simulink model "CLSfixed"  (R2024b)
settings: Solver=FixedStepAuto  StartTime=0.0  StopTime=3000  FixedStep=stepsize  RelTol=1e-3
undefined symbols (not defined in the file or in its folder): AVI, cfg_length, LRI, pNode_length, pPath_length, PVARP, stepsize, URI, VRP
libraries: Libs_unified x311
(part 4 of 4)

== matlab function CLSfixed/Plotting ==
  data: t input; u input
function fcn(t,u)
%coder.extrinsic('evalin')
coder.extrinsic('updateGUIplots')
fun = 'updateGUIplots';
updateGUIplots(t,u)
%feval(fun,t,u)
end

== stateflow chart CLSfixed/cfgs ==
  settings: executeAtInitialization=1
  state Ini
  state wait
  Ini -> wait : [t>800]{pUpdate(Paras);}
  (default) -> Ini : {Sensing=Scfgf;[Monitor, Pre]=Precfg;...
      |  [Heart] =LoadInit;}
  data: Scfg function_output; Mcfg function_output; Preout function_output; LRI parameter; AVI parameter; VRP parameter; URI parameter; PVARP parameter; Parasin function_input; pNode_length parameter; pPath_length parameter; Hcfg function_output; cfg_length parameter; Heart output; Sensing output; Monitor output; t input; Paras input; Pre output
  function Scfg= Scfgf:
    | function Scfg= Scfgf
    | 
    | %% desired
    | xa=1;
    | xc=0.05;
    | xc1=0.1;
    | xd=1;
    | xe=0.1;
    | avd=100;
    | vad=100;
    | uni_a=1;
    | Sens_a=0.6;
    | Amp_ap=500;
    | uni_v=1;
    | Sens_v=2.8;
    | Amp_vp=500;
    | 
    | Scfg=[xa xc xc1 xd xe avd vad uni_a Sens_a Amp_ap uni_v Sens_v Amp_vp]';
    | 
    | end
  function [Mcfg,Preout]= Precfg:
    | function [Mcfg,Preout]= Precfg
    | % 
    | % LRI=1000;
    | % AVI=170;
    | % URI=500;
    | % VRP=230;
    | % PVARP=250;
    | Mcfg=[LRI AVI URI VRP PVARP];
    | Preout=[VRP PVARP];
    | 
    | end
  function pUpdate(Parasin):
    | %% Get the index of the parameter
    | function pUpdate(Parasin)
    | %#codegen
    | coder.extrinsic('evalin');
    | coder.extrinsic('assignin');
    | Nodein=zeros(1,pNode_length); % The total number of cell cfg ports
    | Nodein=evalin('base', 'pNode');
    | Pathin=zeros(1,pPath_length); % The total number of path cfg ports
    | Pathin=evalin('base', 'pPath');
    | for n=1:pNode_length
    |     m=Nodein(n);
    |     Heart(m)=Parasin(n);
    | end
    | 
    | for n=1:pPath_length
    |     m=Pathin(n);
    |     nn=n+length(Nodein);
    |     Heart(m)=Parasin(nn);
    | end
    | 
    | assignin('base', 'Params', Parasin);
    | 
    | end
  function Hcfg   = LoadInit:
    | function Hcfg   = LoadInit
    | %#codegen
    | coder.extrinsic('evalin');
    | Hcfg1=zeros(1,cfg_length); % The total number of cfg ports
    | Hcfg1=evalin('base', 'cfgdata');
    | Hcfg=Hcfg1';
    | end

== matlab function CLSfixed/newparas ==
  data: newparas output; paras_length parameter

function newparas= auto(paras_length)

coder.extrinsic('evalin');
%par_length = evalin('base','paras_length')
newparas=zeros(1,paras_length); % The total number of cell cfg ports
newparas=evalin('base', 'pp');

end

== stateflow chart CLSfixed/savedata ==
  settings: executeAtInitialization=1
  state termi
  state difa
  state Ini
  difa -> termi [order 1] : [rate_ave_a0>=60]/{coder.extrinsic('assignin');diffa=rate_ave_a1-rate_ave_a0;assignin('base', 'diffa', diffa);}
  (default) -> Ini : {rate_ave_vp=0; diffa=0;smax=0;}
  Ini -> difa [order 1] : [t>=29998]{coder.extrinsic('assignin','mean');assignin('base', 'reqqn', reqqn);assignin('base', 'errn', errn);assignin('base', 'smax', smax);...
      | assignin('base', 'errs', errs);assignin('base', 'reqs', reqs);assignin('base', 'reqqs', reqqs);...
      | assignin('base', 'nas0', nas0);assignin('base', 'nap0', nap0);assignin('base', 'nvs0', nvs0);assignin('base', 'nvp0', nvp0);...
      | assignin('base', 'rate_as0', rate_as0);assignin('base', 'rate_ap0', rate_ap0);assignin('base', 'rate_vs0', rate_vs0);assignin('base', 'rate_vp0', rate_vp0);...
      | assignin('base', 'nas1', nas1);assignin('base', 'nap1', nap1);assignin('base', 'nvs1', nvs1);assignin('base', 'nvp1', nvp1);...
      | assignin('base', 'rate_as1', rate_as1);assignin('base', 'rate_ap1', rate_ap1);assignin('base', 'rate_vs1', rate_vs1);assignin('base', 'rate_vp1', rate_vp1);...
      | rate_ave_vp=mean(rate_vp1(2,1:nvp1));assignin('base', 'rate_ave_vp', rate_ave_vp);...
      | rate_ave_a1=0;rate_ave_a1=mean([rate_as1(2,1:nas1) ]);rate_ave_a0=0;rate_ave_a0=mean(rate_as0(2,1:nas0));}
  difa -> termi [order 2] : [rate_ave_a0<60]/{coder.extrinsic('assignin');diffa=rate_ave_a1-60;assignin('base', 'diffa', diffa);}
  Ini -> Ini [order 2] : [s>smax]/{smax=s;}
  data: t input; reqqn input; errn input; s input; reqs input; errs input; reqqs input; nas0 input; nap0 input; nvs0 input; nvp0 input; rate_as0 input; rate_ap0 input; rate_vs0 input; rate_vp0 input; nas1 input; nap1 input; nvs1 input; nvp1 input; rate_as1 input; rate_ap1 input; rate_vs1 input; rate_vp1 input; diffa output double; rate_ave_a1 local double; rate_ave_vp output double; rate_ave_a0 local double; smax local
